simulink model "EjercicioResueltoSimulink"  (R2018a)
settings: Solver=ode4  StartTime=0.0  StopTime=30  FixedStep=1e-4  MinStep=1e-6  RelTol=1e-3
settings Model: Creator=Fondecyt 3170897  LastModifiedBy=Fondecyt 3170897

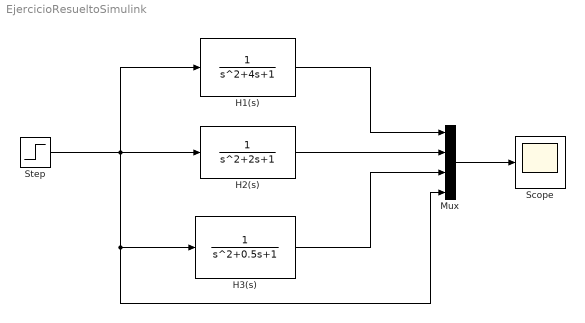
== system EjercicioResueltoSimulink ==
  H1(s) : TransferFcn  Denominator=[1 4 1]
  H2(s) : TransferFcn
  H3(s) : TransferFcn  Denominator=[1 0.5 1]
  Mux : Mux
  Scope : Scope
  Step : Step  SampleTime=0
  wires:
  Step/1 -> H3(s)/1, Mux/4, H2(s)/1, H1(s)/1
  H1(s)/1 -> Mux/1
  H2(s)/1 -> Mux/2
  H3(s)/1 -> Mux/3
  Mux/1 -> Scope/1
